simulink model "HalfBridgeCapacitanceModellin"  (R2016a)
settings: Solver=FixedStepDiscrete  StartTime=0.0  StopTime=3e-6  RelTol=1e-3
values from neighbouring files (symbols this model uses):
  Dbot = 49    [HalfBridge.m]    (also in HalfBridgeBottomConnectedLoad.m; HalfBridgeCapacitanceModelling.m)
  DelayBot = 0    [HalfBridge.m]    (also in HalfBridgeBottomConnectedLoad.m = 50; HalfBridgeCapacitanceModelling.m = 50)
  DelayTop = 50    [HalfBridge.m]    (also in HalfBridgeBottomConnectedLoad.m = 0; HalfBridgeCapacitanceModelling.m = 0)
  Dtop = 49    [HalfBridge.m]    (also in HalfBridgeBottomConnectedLoad.m; HalfBridgeCapacitanceModelling.m)
  fsw = 1e6    (= 1000000)    [ChannelAndDSTrajectories.m]    (also in GanModel_Nonsegmented.m = 100000; HalfBridge.m; HalfBridgeBottomConnectedLoad.m; HalfBridgeCapacitanceModelling.m)
  Rd = 3.6*0.95*0.82*18.2*0.25/295    (= 0.0432543050847)    [AnalyticalModel.m]    (also in GanModel_Nonsegmented.m = 0.1; HalfBridge.m = 2.5e-05; HalfBridgeBottomConnectedLoad.m = 2.5e-05; HalfBridgeCapacitanceModelling.m = 2.5e-05)
  Rg = 1    [GanModel_Nonsegmented.m]    (also in HalfBridge.m; HalfBridgeBottomConnectedLoad.m = 1.5; HalfBridgeCapacitanceModelling.m = 1.5)
  Rload = 10    [GanModel_Nonsegmented.m]    (also in HalfBridge.m; HalfBridgeBottomConnectedLoad.m; HalfBridgeCapacitanceModelling.m = 13.3333333333)
  Roff = 2    [HalfBridge.m]    (also in HalfBridgeBottomConnectedLoad.m; HalfBridgeCapacitanceModelling.m = 5)
  Ron = 12    [HalfBridge.m]    (also in HalfBridgeBottomConnectedLoad.m; HalfBridgeCapacitanceModelling.m = 20)
  Rs = 3.6*0.238*0.82/295    (= 0.00238161355932)    [AnalyticalModel.m]    (also in GanModel_Nonsegmented.m = 0.1; HalfBridge.m = 2.5e-05; HalfBridgeBottomConnectedLoad.m = 2.5e-05; HalfBridgeCapacitanceModelling.m = 2.5e-05)
libraries: elec_lib x36, nesl_utility x27, fl_lib x21
(part 2 of 2)

== matlab function HalfBridgeCapacitanceModellin/GaN_Bot/MATLAB Function ==
  data: Vgs input; Ids output; Vds input
function Ids = fcn(Vgs,Vds)
%#codegen
% K1 = 0.283;
% b1 = 2.035;
% c1 = 0.124;
% d1 = 1.159;
% e1 = -0.204;
% m1 = 30.972;
% n1 = -4.48;
% K2 = 7.114;
% b2 = 2.054;
% c2 = 0.153;
Vgd = Vgs - Vds;

cur = 4.5057;
K = cur * 0.8 * (273/300)^(-2.7);
x0 = 0.31 ;
x1 = 0.255;
slp = 2;


% if Vds>0
%     Ids = K1*log(1+exp((Vgs-b1)/c1))*((m1+n1*Vgs)*Vds)/(1+(d1+e1*Vgs)*Vds);
% else
% 
%     Ids = -K2*log(1+exp((Vgd-b2)/c2))*(-Vds/(1-Vds));
% end

if Vds>0
    Ids = K*log(1+exp(26*(Vgs-1.7)/slp))*(Vds)/(1+max((x0+x1*(Vgs+4.1)),0.2)*Vds);
else

    Ids = -K*log(1+exp(21*(Vgd-1.7)/slp))*(-Vds)/(1+max((x0+x1*(Vgd+6.1)),0.2)*(-Vds));
end

== matlab function HalfBridgeCapacitanceModellin/GaN_Top/MATLAB Function ==
  data: Vgs input; Ids output; Vds input
function Ids = fcn(Vgs,Vds)
%#codegen
% K1 = 0.283;
% b1 = 2.035;
% c1 = 0.124;
% d1 = 1.159;
% e1 = -0.204;
% m1 = 30.972;
% n1 = -4.48;
% K2 = 7.114;
% b2 = 2.054;
% c2 = 0.153;
Vgd = Vgs - Vds;

cur = 4.5057;
K = cur * 0.8 * (273/300)^(-2.7);
x0 = 0.31 ;
x1 = 0.255;
slp = 2;


% if Vds>0
%     Ids = K1*log(1+exp((Vgs-b1)/c1))*((m1+n1*Vgs)*Vds)/(1+(d1+e1*Vgs)*Vds);
% else
% 
%     Ids = -K2*log(1+exp((Vgd-b2)/c2))*(-Vds/(1-Vds));
% end

if Vds>0
    Ids = K*log(1+exp(26*(Vgs-1.7)/slp))*(Vds)/(1+max((x0+x1*(Vgs+4.1)),0.2)*Vds);
else

    Ids = -K*log(1+exp(21*(Vgd-1.7)/slp))*(-Vds)/(1+max((x0+x1*(Vgd+6.1)),0.2)*(-Vds));
end

== matlab function HalfBridgeCapacitanceModellin/GaN_Top/Capacitance Calculator/MATLAB Function ==
  data: Vds input; Cgs output; Cgd output; Cds output
function [Cgs,Cgd,Cds]= fcn(Vds)
%#codegen
Vds = abs(Vds);
%% Crss calculation
       a1 =   2.519e+14;
       b1 =      -345.7;
       c1 =       63.76;
       a2 =       27.99;
       b2 =       12.86;
       c2 =       18.29;
       a3 =       8.666;
       b3 =       33.93;
       c3 =       9.161;
       a4 =       1.502;
       b4 =       125.5;
       c4 =       121.9;
       a5 =      0.6563;
       b5 =         500;
       c5 =       34.57;
       a6 =        1.98;
       b6 =       408.2;
       c6 =       134.7;
Crss = a1.*exp(-((Vds-b1)./c1).^2) + a2.*exp(-((Vds-b2)./c2).^2) + a3*exp(-((Vds-b3)./c3).^2)...
   + a4.*exp(-((Vds-b4)./c4).^2) +a5.*exp(-((Vds-b5)./c5).^2) +a6.*exp(-((Vds-b6)./c6).^2);
Crss = Crss*1e-12;
%% Ciss Calculation
       a1 =        1167;
       b1 =      -115.8;
       c1 =       60.96;
       a2 =       269.7;
       b2 =       -5402;
       c2 =   4.243e+04;
       a3 =        3.61;
       b3 =       238.5;
       c3 =       2.507;
       a4 =       1.036;
       b4 =       175.8;
       c4 =       16.81;
       a5 =       1.571;
       b5 =         263;
       c5 =       3.586;
       a6 =      -1.174;
       b6 =       238.2;
       c6 =       25.85;
Ciss = a1.*exp(-((Vds-b1)./c1).^2) + a2.*exp(-((Vds-b2)./c2).^2) + a3*exp(-((Vds-b3)./c3).^2)...
   + a4.*exp(-((Vds-b4)./c4).^2) +a5.*exp(-((Vds-b5)./c5).^2) +a6.*exp(-((Vds-b6)./c6).^2);
Ciss = Ciss*1e-12;
%% Coss Calculation
       a1 =         328;
       b1 =       -8.43;
       c1 =       30.26;
       a2 =       115.8;
       b2 =        42.2;
       c2 =       7.341;
       a3 =       45.83;
       b3 =       59.01;
       c3 =       6.099;
       a4 =       183.1;
       b4 =        28.6;
       c4 =       16.39;
       a5 =       69.29;
       b5 =       154.4;
       c5 =        1511;
       a6 =       125.6;
       b6 =       22.68;
       c6 =       119.6;
Coss = a1.*exp(-((Vds-b1)./c1).^2) + a2.*exp(-((Vds-b2)./c2).^2) + a3*exp(-((Vds-b3)./c3).^2)...
   + a4.*exp(-((Vds-b4)./c4).^2) +a5.*exp(-((Vds-b5)./c5).^2) +a6.*exp(-((Vds-b6)./c6).^2);
Coss = Coss*1e-12;
%% Outputs
Cgs = Ciss - Crss;
Cds = Coss - Crss;
Cgd = Crss;

== matlab function HalfBridgeCapacitanceModellin/GaN_Bot/Capacitance Calculator/MATLAB Function ==
  data: Vds input; Cgs output; Cgd output; Cds output
function [Cgs,Cgd,Cds]= fcn(Vds)
%#codegen
Vds = abs(Vds);
%% Crss calculation
       a1 =   2.519e+14;
       b1 =      -345.7;
       c1 =       63.76;
       a2 =       27.99;
       b2 =       12.86;
       c2 =       18.29;
       a3 =       8.666;
       b3 =       33.93;
       c3 =       9.161;
       a4 =       1.502;
       b4 =       125.5;
       c4 =       121.9;
       a5 =      0.6563;
       b5 =         500;
       c5 =       34.57;
       a6 =        1.98;
       b6 =       408.2;
       c6 =       134.7;
Crss = a1.*exp(-((Vds-b1)./c1).^2) + a2.*exp(-((Vds-b2)./c2).^2) + a3*exp(-((Vds-b3)./c3).^2)...
   + a4.*exp(-((Vds-b4)./c4).^2) +a5.*exp(-((Vds-b5)./c5).^2) +a6.*exp(-((Vds-b6)./c6).^2);
Crss = Crss*1e-12;
%% Ciss Calculation
       a1 =        1167;
       b1 =      -115.8;
       c1 =       60.96;
       a2 =       269.7;
       b2 =       -5402;
       c2 =   4.243e+04;
       a3 =        3.61;
       b3 =       238.5;
       c3 =       2.507;
       a4 =       1.036;
       b4 =       175.8;
       c4 =       16.81;
       a5 =       1.571;
       b5 =         263;
       c5 =       3.586;
       a6 =      -1.174;
       b6 =       238.2;
       c6 =       25.85;
Ciss = a1.*exp(-((Vds-b1)./c1).^2) + a2.*exp(-((Vds-b2)./c2).^2) + a3*exp(-((Vds-b3)./c3).^2)...
   + a4.*exp(-((Vds-b4)./c4).^2) +a5.*exp(-((Vds-b5)./c5).^2) +a6.*exp(-((Vds-b6)./c6).^2);
Ciss = Ciss*1e-12;

%% Coss Calculation
       a1 =         328;
       b1 =       -8.43;
       c1 =       30.26;
       a2 =       115.8;
       b2 =        42.2;
       c2 =       7.341;
       a3 =       45.83;
       b3 =       59.01;
       c3 =       6.099;
       a4 =       183.1;
       b4 =        28.6;
       c4 =       16.39;
       a5 =       69.29;
       b5 =       154.4;
       c5 =        1511;
       a6 =       125.6;
       b6 =       22.68;
       c6 =       119.6;
Coss = a1.*exp(-((Vds-b1)./c1).^2) + a2.*exp(-((Vds-b2)./c2).^2) + a3*exp(-((Vds-b3)./c3).^2)...
   + a4.*exp(-((Vds-b4)./c4).^2) +a5.*exp(-((Vds-b5)./c5).^2) +a6.*exp(-((Vds-b6)./c6).^2);
Coss = Coss*1e-12;
%% Outputs
Cgs = Ciss - Crss;
Cds = Coss - Crss;
Cgd = Crss;
